simulink model "VerificaEIG"  (R2025b)
settings: Solver=VariableStepAuto  StartTime=0.0  StopTime=10.0  RelTol=1e-3
values from neighbouring files (symbols this model uses):
  A = double(subs(A_sym, p_eq_instabile, val_instabili))    [SvolgimentoEsame.m]
  B = double(subs(B_sym, p_eq_instabile, val_instabili))    [SvolgimentoEsame.m]
  C = eye(4)    [SvolgimentoEsame.m]
  D = zeros(4, 1)    [SvolgimentoEsame.m]
  K_2 = place(A, B, p)    [SvolgimentoEsame.m]
  X_initial = [x0; dx0; th0; dth0]    [SvolgimentoEsame.m]
settings Model: Creator=salvo  LastModifiedBy=salvo

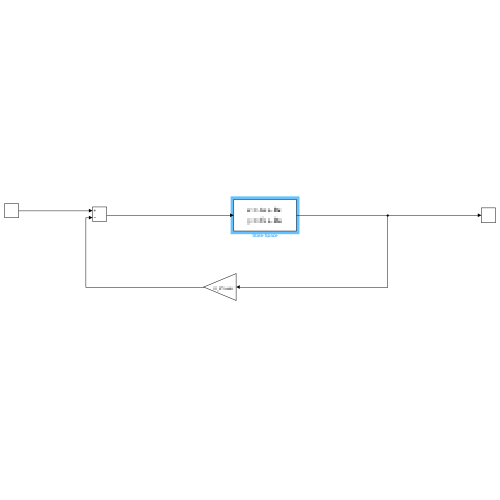
[thumbnail: Simulink's stored preview of the top-level diagram]
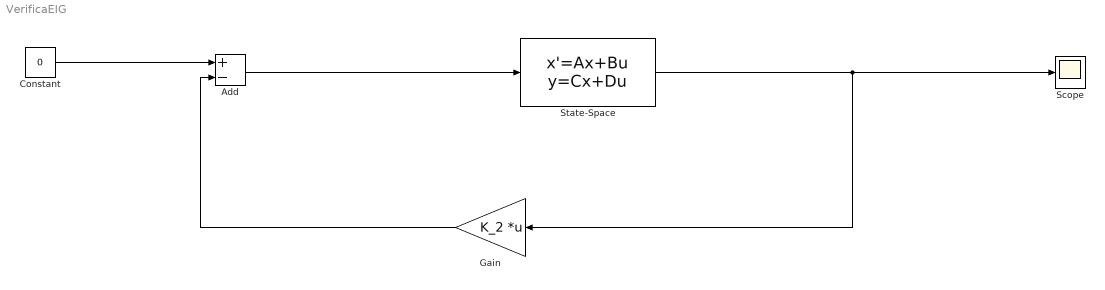
== system VerificaEIG ==
  Add : Sum  Inputs=+-
  Constant : Constant  Value=0
  Gain : Gain  Gain=K_2  Multiplication=Matrix(K*u) (u vector)
  Scope : Scope
      settings: ActiveDisplayYMinimum=-6.8016594835568576  ActiveDisplayYMaximum=7.7694776313724478
  State-Space : StateSpace  A=A  B=B  C=C  D=D  InitialCondition=X_initial
  wires:
  Gain/1 -> Add/2
  Add/1 -> State-Space/1
  State-Space/1 -> Scope/1, Gain/1
  Constant/1 -> Add/1
